simulink model "vehicle_indicators_fsm"  (R2019a)
settings: Solver=FixedStepDiscrete  StartTime=0.0  StopTime=3  RelTol=1e-3
settings Model: Creator=penum  LastModifiedBy=penum
settings OptimizationCC: DefaultParameterBehavior=Inlined  UseDivisionForNetSlopeComputation=on  GainParamInheritBuiltInType=on  UseFloatMulNetSlope=on  InlineInvariantSignals=on  PassReuseOutputArgsAs=Individual arguments  ZeroExternalMemoryAtStartup=off  ZeroInternalMemoryAtStartup=off  NoFixptDivByZeroProtection=on  EfficientFloat2IntCast=on  LifeSpan=1  OptimizeBlockOrder=speed  DifferentSizesBufferReuse=on
settings DebuggingCC: ParameterTunabilityLossMsg=error
settings HardwareCC: ProdBitPerInt=16  ProdBitPerPointer=16  ProdBitPerSizeT=16  ProdBitPerPtrDiffT=16  ProdLargestAtomicFloat=None  ProdWordSize=16  ProdLongLongMode=on  ProdHWDeviceType=Atmel->AVR (8-bit)
settings SFSimCC: MATLABDynamicMemAlloc=off
settings RTWCC: SystemTargetFile=ert.tlc  TemplateMakefile=ert_default_tmf  GenerateReport=on  IncludeHyperlinkInReport=on  LaunchReport=on  GenerateTraceInfo=on  GenerateTraceReport=on  GenerateTraceReportSl=on  GenerateTraceReportSf=on  GenerateTraceReportEml=on  GenerateCodeMetricsReport=on
settings CodeAppCC: ForceParamTrailComments=on  IgnoreCustomStorageClasses=off  OperatorAnnotations=on  SimulinkDataObjDesc=on  SFDataObjDesc=on  CustomSymbolStrGlobalVar=rt$N$M  CustomSymbolStrType=$N$M  CustomSymbolStrFcn=$N$M$F  CustomSymbolStrMacro=$N$M  InsertBlockDesc=on
settings ERTTargetCC: TargetLangStandard=C99 (ISO)  GenerateSampleERTMain=on  IncludeMdlTerminateFcn=off  CombineSignalStateStructs=on  SupportAbsoluteTime=off  SupportComplex=off  SupportNonInlinedSFcns=on  InlinedParameterPlacement=NonHierarchical  RootIOFormat=Structure reference  ERTCustomFileTemplate=example_file_process.tlc  ERTFilePackagingFormat=CompactWithDataFile

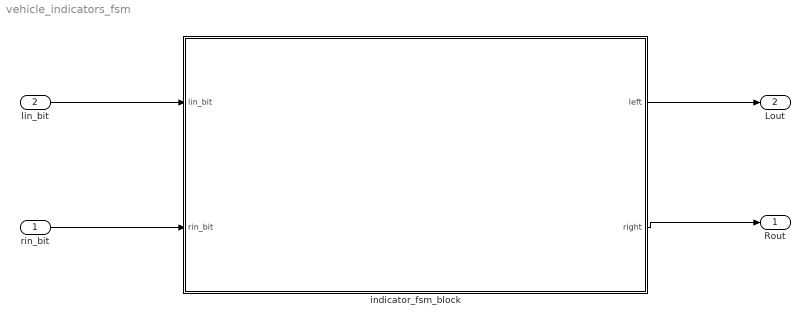
== system vehicle_indicators_fsm ==
  rin_bit : Inport
  lin_bit : Inport  Port=2
  indicator_fsm_block : Stateflow chart  BlockKeywords=__PRM__SERIALIZED__DATA__:Stateflow Chart,Stateflow Diagram  TreatAsAtomicUnit=on
  Rout : Outport
  Lout : Outport  Port=2
  wires:
  indicator_fsm_block/2(right) -> Rout/1
  rin_bit/1 -> indicator_fsm_block/2(rin_bit)
  lin_bit/1 -> indicator_fsm_block/1(lin_bit)
  indicator_fsm_block/1(left) -> Lout/1

== stateflow chart vehicle_indicators_fsm/indicator_fsm_block ==
  state BothON
    entry, during:
    left=1;
    right=1;
    count = 0;
  state Count
    entry, during:
    left=0;
    right=0;
    count = count + 1;
  state LeftON
    entry:
    left=double(not(left));
    right=0;
    count = 0;
  state OFF
    entry, during:
    left=0;
    right=0;
    count=0;
  state RightON
    entry:
    left=0;
    right=double(not(right));
    count = 0;
  (junction 29) -> Count
  (junction 18) -> BothON [order 1] : [(lin_bit == 1) & (rin_bit == 1)]
  BothON -> (junction 29) : [(lin_bit == 1) | (rin_bit == 1)]
  (default) -> OFF : {count=0;}
  OFF -> Count : [(lin_bit == 1) | (rin_bit == 1)]
  LeftON -> (junction 29) : [(lin_bit == 1) | (rin_bit == 1)]
  RightON -> (junction 29) : [(lin_bit == 1) | (rin_bit == 1)]
  Count -> (junction 18) [order 2] : [count==10]
  (junction 18) -> LeftON [order 2] : [lin_bit == 1]
  (junction 18) -> RightON [order 3] : [rin_bit == 1]
  Count -> OFF [order 1] : [(lin_bit == 0) & (rin_bit == 0)]
  data: lin_bit input size=1; rin_bit input size=1; left output size=1 =0; right output size=1 =0; count local
